simulink model "model_tmp_1p"  (R2015b)
settings: Solver=ode15s  StartTime=0.0  StopTime=T_sim  FixedStep=dt  RelTol=1e-3
PreLoadFcn:
  | setup_tmp_1p;
InitFcn:
  | setup_tmp_1p;
values from neighbouring files (symbols this model uses):
  A_act = [-100 0 0 0 0 -100 0 0 0 0 -100 0 ... (16 elements, 4x4)]    [CD_spline.mat]    (also in CL_spline.mat; setup.m = -100*eye(4); setup_tmp_1p.m = -100*eye(4); setup_tmp_4p.m = -100*eye(4))
  A_Kite = 7    [CD_spline.mat]    (also in CL_spline.mat; setup.m = 10.18; setup_tmp_1p.m = 10.18; setup_tmp_4p.m = 10.18)
  A_prd = [0 0 0 -640 0 0 0 0 0 0 -640 0 ... (36 elements, 6x6)]    [CD_spline.mat]    (also in CL_spline.mat; setup.m = 1000 * A_M_aug; setup_tmp_1p.m = 1000 * A_M_aug; setup_tmp_4p.m = 1000 * A_M_aug)
  A_ref = [0 0 0 -10000 0 0 0 0 0 0 -10000 0 ... (36 elements, 6x6)]    [CD_spline.mat]    (also in CL_spline.mat; setup.m = zeros(6); setup_tmp_1p.m = zeros(6); setup_tmp_4p.m = zeros(6))
  A_t_ref_cl = [0 0 0 -0.64 0 0 0 0 0 0 -0.64 0 ... (36 elements, 6x6)]    [CD_spline.mat]    (also in CL_spline.mat; setup.m = A_t_ref; setup_tmp_1p.m = A_t_ref; setup_tmp_4p.m = A_t_ref)
  ASideRel = 0    [CD_spline.mat]    (also in CL_spline.mat; setup.m; setup_tmp_1p.m; setup_tmp_4p.m)
  B_act = [100 0 0 0 0 100 0 0 0 0 100 0 ... (16 elements, 4x4)]    [CD_spline.mat]    (also in CL_spline.mat; setup.m = 100*eye(4); setup_tmp_1p.m = 100*eye(4); setup_tmp_4p.m = 100*eye(4))
  B_ref = [0 0 0 10000 0 0 0 0 0 0 10000 0 ... (18 elements, 6x3)]    [CD_spline.mat]    (also in CL_spline.mat; setup.m = zeros(6,3); setup_tmp_1p.m = zeros(6,3); setup_tmp_4p.m = zeros(6,3))
  B_t_ref_cl = [0 0 0 0.64 0 0 0 0 0 0 0.64 0 ... (18 elements, 6x3)]    [CD_spline.mat]    (also in CL_spline.mat)
  Bpbl = [0 0 0 1 0 0 0 0 0 0 1 0 ... (18 elements, 6x3)]    [CD_spline.mat]    (also in CL_spline.mat; setup.m = [zeros(3); eye(3)]; setup_tmp_1p.m = [zeros(3); eye(3)]; setup_tmp_4p.m = [zeros(3); eye(3)])
  c0 = 614000    [CD_spline.mat]    (also in CL_spline.mat; setup.m; setup_tmp_1p.m; setup_tmp_4p.m)
  C_A = [0 0.3 -1e-06 1 -0.3 0 1e-06 1 0 -0.3 -1e-06 1 ... (16 elements, 4x4)]    [CD_spline.mat]    (also in CL_spline.mat; setup.m = [0, -R, 0, R; setup_tmp_1p.m = [0, -R, 0, R; setup_tmp_4p.m = [0, -R, 0, R)
  C_A_inv = [0 -1.66666666667 -1.23358113847e-17 1.66666666667 1.66666666667 2.46716227694e-17 -1.66666666667 0 -250000 250000 -250000 250000 ... (16 elements, 4x4)]    [CD_spline.mat]    (also in CL_spline.mat; setup.m = C_A \eye(4); setup_tmp_1p.m = C_A \eye(4); setup_tmp_4p.m = C_A \eye(4))
  C_D_Kite = 0.05    [CD_spline.mat]    (also in CL_spline.mat; setup.m = 0.005; setup_tmp_1p.m = 0.005; setup_tmp_4p.m = 0.005)
  C_L_Kite = 0.1    [CD_spline.mat]    (also in CL_spline.mat; setup.m = 0.01; setup_tmp_1p.m = 0.01; setup_tmp_4p.m = 0.01)
  CD_tether = 0.96    [CD_spline.mat]    (also in CL_spline.mat; setup.m; setup_tmp_1p.m; setup_tmp_4p.m)
  d0 = 473    [CD_spline.mat]    (also in CL_spline.mat; setup.m; setup_tmp_1p.m; setup_tmp_4p.m)
  d_tether = 0.004    [CD_spline.mat]    (also in CL_spline.mat; setup.m; setup_tmp_1p.m; setup_tmp_4p.m)
  delta_dead = 0.5    [CD_spline.mat]    (also in CL_spline.mat; setup.m; setup_tmp_1p.m; setup_tmp_4p.m)
  e_0 = 0.01    [CD_spline.mat]    (also in CL_spline.mat; setup.m; setup_tmp_1p.m; setup_tmp_4p.m)
  epsilon = 0.6    [CD_spline.mat]    (also in CL_spline.mat; setup.m; setup_tmp_1p.m; setup_tmp_4p.m)
  eta_init = [0 0 0]    [CD_spline.mat]    (also in CL_spline.mat; setup.m = zeros(3,1); setup_tmp_1p.m = zeros(3,1); setup_tmp_4p.m = zeros(3,1))
  g = 9.81    [CD_spline.mat]    (also in CL_spline.mat; setup.m; setup_tmp_1p.m; setup_tmp_4p.m)
  g_vec = [0 0 9.81]    [CD_spline.mat]    (also in CL_spline.mat; setup.m = [0;0;9.81]; setup_tmp_1p.m = [0;0;9.81]; setup_tmp_4p.m = [0;0;9.81])
  Gamma_ad = 100    [CD_spline.mat]    (also in CL_spline.mat; setup.m = 100;100; setup_tmp_1p.m = 100;100; setup_tmp_4p.m = 100;100)
  Gamma_pred = 100    [CD_spline.mat]    (also in CL_spline.mat; setup.m; setup_tmp_1p.m; setup_tmp_4p.m)
  J = [0.018  0  0; 0  0.018  0; 0  0  0.009]    [CD_spline.mat]    (also in CL_spline.mat; setup.m = diag([Ixx, Iyy, Izz]); setup_tmp_1p.m = diag([Ixx, Iyy, Izz]); setup_tmp_4p.m = diag([Ixx, Iyy, Izz]))
  Jinv = [55.5555555556  0  0; 0  55.5555555556  0; 0  0  111.111111111]    [CD_spline.mat]    (also in CL_spline.mat; setup.m = J \ eye(3); setup_tmp_1p.m = J \ eye(3); setup_tmp_4p.m = J \ eye(3))
  k_e_eta = 10000    [CD_spline.mat]    (also in CL_spline.mat; setup.m; setup_tmp_1p.m; setup_tmp_4p.m)
  k_e_eta_dot = 400    [CD_spline.mat]    (also in CL_spline.mat; setup.m; setup_tmp_1p.m; setup_tmp_4p.m)
  k_e_eta_I = 1    [CD_spline.mat]    (also in CL_spline.mat; setup.m; setup_tmp_1p.m; setup_tmp_4p.m)
  K_i_t = [10  0  0; 0  10  0; 0  0  10]    [CD_spline.mat]    (also in CL_spline.mat; setup.m = 10*eye(3); setup_tmp_1p.m = 10*eye(3); setup_tmp_4p.m = 10*eye(3))
  K_v_t = [1.6  0  0; 0  1.6  0; 0  0  1.6]    [CD_spline.mat]    (also in CL_spline.mat; setup.m = 2*omega_0_trans*zeta_0_trans*eye(3); setup_tmp_1p.m = 2*omega_0_trans*zeta_0_trans*eye(3); setup_tmp_4p.m = 2*omega_0_trans*zeta_0_trans*eye(3))
  K_x_t = [0.64  0  0; 0  0.64  0; 0  0  0.64]    [CD_spline.mat]    (also in CL_spline.mat; setup.m = omega_0_trans^2*eye(3); setup_tmp_1p.m = omega_0_trans^2*eye(3); setup_tmp_4p.m = omega_0_trans^2*eye(3))
  l_s0 = 1    [CD_spline.mat]    (also in CL_spline.mat; setup.m = 1.42857142857; setup_tmp_1p.m = 1.42857142857; setup_tmp_4p.m = 2)
  m_kite = 7    [CD_spline.mat]    (also in CL_spline.mat; setup.m; setup_tmp_1p.m = 5;7; setup_tmp_4p.m = 6.21)
  m_p = 0.013    [CD_spline.mat]    (also in CL_spline.mat; setup.m = 0.0185714285714; setup_tmp_1p.m = 0.0185714285714; setup_tmp_4p.m = 0.026)
  m_uav = 3    [CD_spline.mat]    (also in CL_spline.mat; setup.m; setup_tmp_1p.m; setup_tmp_4p.m)
  n = 10    [CD_spline.mat]    (also in CL_spline.mat; setup.m; setup_tmp_1p.m; setup_tmp_4p.m)
  omega_init = [0 0 0]    [CD_spline.mat]    (also in CL_spline.mat; setup.m = zeros(3,1); setup_tmp_1p.m = zeros(3,1); setup_tmp_4p.m = zeros(3,1))
  p_init = [0 0 1 0 0 2 0 0 3 0 0 4 ... (30 elements, 30x1)]    [CD_spline.mat]    (also in CL_spline.mat; setup.m = zeros(3*n,1); setup_tmp_1p.m = zeros(3*n,1); setup_tmp_4p.m = zeros(3*n,1))
  P_prd = [712.5 0 0 156.25 0 0 0 712.5 0 0 156.25 0 ... (36 elements, 6x6)]    [CD_spline.mat]    (also in CL_spline.mat; setup.m = 1000 * P_tref; setup_tmp_1p.m = 1000 * P_tref; setup_tmp_4p.m = 1000 * P_tref)
  P_tref = [0.7125 0 0 0.15625 0 0 0 0.7125 0 0 0.15625 0 ... (36 elements, 6x6)]    [CD_spline.mat]    (also in CL_spline.mat; setup.m = lyap(A_M_aug', Q); setup_tmp_1p.m = lyap(A_M_aug', Q); setup_tmp_4p.m = lyap(A_M_aug', Q))
  rho_air = 1.225    [CD_spline.mat]    (also in CL_spline.mat; setup.m; setup_tmp_1p.m; setup_tmp_4p.m)
  rho_t = 0.013    [CD_spline.mat]    (also in CL_spline.mat; setup.m; setup_tmp_1p.m; setup_tmp_4p.m)
  sample_log = 0.01    [CD_spline.mat]    (also in CL_spline.mat; setup.m; setup_tmp_1p.m; setup_tmp_4p.m)
  t0 = 1    [CD_spline.mat]    (also in CL_spline.mat; setup.m; setup_tmp_1p.m; setup_tmp_4p.m)
  t1 = 3    [CD_spline.mat]    (also in CL_spline.mat; setup.m; setup_tmp_1p.m; setup_tmp_4p.m)
  T_launch = 40    [CD_spline.mat]    (also in CL_spline.mat; setup.m; setup_tmp_1p.m; setup_tmp_4p.m)
  Theta_max = 60    [CD_spline.mat]    (also in CL_spline.mat; setup.m; setup_tmp_1p.m; setup_tmp_4p.m)
  Thrust_Max = 80    [CD_spline.mat]    (also in CL_spline.mat; setup.m; setup_tmp_1p.m = 100; setup_tmp_4p.m = 1000000000)
  Tx = 10    [CD_spline.mat]    (also in CL_spline.mat; setup.m; setup_tmp_1p.m; setup_tmp_4p.m)
  Ty = 10    [CD_spline.mat]    (also in CL_spline.mat; setup.m; setup_tmp_1p.m; setup_tmp_4p.m)
  Tz = 10    [CD_spline.mat]    (also in CL_spline.mat; setup.m; setup_tmp_1p.m; setup_tmp_4p.m)
  v_w_vec = [1 1 1]    [CD_spline.mat]    (also in CL_spline.mat; setup.m = [1;0;0]; setup_tmp_1p.m = [1;0;0]; setup_tmp_4p.m = [1;0;0])
  x0num = 0    [CD_spline.mat]    (also in CL_spline.mat; polynomial_trajectory.m = double( solutions_x.x0 ))
  x1num = 0    [CD_spline.mat]    (also in CL_spline.mat; polynomial_trajectory.m = double( solutions_x.x1 ))
  x2num = 0    [CD_spline.mat]    (also in CL_spline.mat; polynomial_trajectory.m = double( solutions_x.x2 ))
  x3num = 0.05    [CD_spline.mat]    (also in CL_spline.mat; polynomial_trajectory.m = double( solutions_x.x3 ))
  x4num = -0.0075    [CD_spline.mat]    (also in CL_spline.mat; polynomial_trajectory.m = double( solutions_x.x4 ))
  x5num = 0.0003    [CD_spline.mat]    (also in CL_spline.mat; polynomial_trajectory.m = double( solutions_x.x5 ))
  x_drone_init = [0 0 10]    [CD_spline.mat]    (also in CL_spline.mat; setup.m = p_init(3*n-2:3*n); setup_KiteModel_4points.m = pos_UAV_init; setup_tmp_1p.m = p_init(3*n-2:3*n))
  xT = 5    [CD_spline.mat]    (also in CL_spline.mat; setup.m; setup_tmp_1p.m = 10; setup_tmp_4p.m = 10)
  y0num = 0    [CD_spline.mat]    (also in CL_spline.mat; polynomial_trajectory.m = double( solutions_y.y0 ))
  y1num = 0    [CD_spline.mat]    (also in CL_spline.mat; polynomial_trajectory.m = double( solutions_y.y1 ))
  y2num = 0    [CD_spline.mat]    (also in CL_spline.mat; polynomial_trajectory.m = double( solutions_y.y2 ))
  y3num = 0.1    [CD_spline.mat]    (also in CL_spline.mat; polynomial_trajectory.m = double( solutions_y.y3 ))
  y4num = -0.015    [CD_spline.mat]    (also in CL_spline.mat; polynomial_trajectory.m = double( solutions_y.y4 ))
  y5num = 0.0006    [CD_spline.mat]    (also in CL_spline.mat; polynomial_trajectory.m = double( solutions_y.y5 ))
  yT = 10    [CD_spline.mat]    (also in CL_spline.mat; setup.m; setup_tmp_1p.m = 0; setup_tmp_4p.m = 0)
  z0num = 10    [CD_spline.mat]    (also in CL_spline.mat; polynomial_trajectory.m = double( solutions_z.z0 ))
  z1num = 0    [CD_spline.mat]    (also in CL_spline.mat; polynomial_trajectory.m = double( solutions_z.z1 ))
  z2num = 0    [CD_spline.mat]    (also in CL_spline.mat; polynomial_trajectory.m = double( solutions_z.z2 ))
  z3num = 0.4    [CD_spline.mat]    (also in CL_spline.mat; polynomial_trajectory.m = double( solutions_z.z3 ))
  z4num = -0.06    [CD_spline.mat]    (also in CL_spline.mat; polynomial_trajectory.m = double( solutions_z.z4 ))
  z5num = 0.0024    [CD_spline.mat]    (also in CL_spline.mat; polynomial_trajectory.m = double( solutions_z.z5 ))
  zT = 50    [CD_spline.mat]    (also in CL_spline.mat; setup.m; setup_tmp_1p.m; setup_tmp_4p.m)
libraries: simulink x1
(part 1 of 2)
settings Model: Creator=Sebastian  LastModifiedBy=srapp
settings OptimizationCC: DefaultParameterBehavior=Inlined
settings DebuggingCC: MultiTaskRateTransMsg=warning
settings HardwareCC: ProdBitPerLong=64  ProdLargestAtomicFloat=None  ProdHWDeviceType=Intel->x86-64  TargetBitPerLong=64  TargetBitPerPointer=64  TargetIntDivRoundTo=Zero  TargetEndianess=LittleEndian  TargetWordSize=64  TargetHWDeviceType=Intel->x86-64
settings RTWCC: RTWCompilerOptimization=on
settings CodeAppCC: MaxIdLength=95

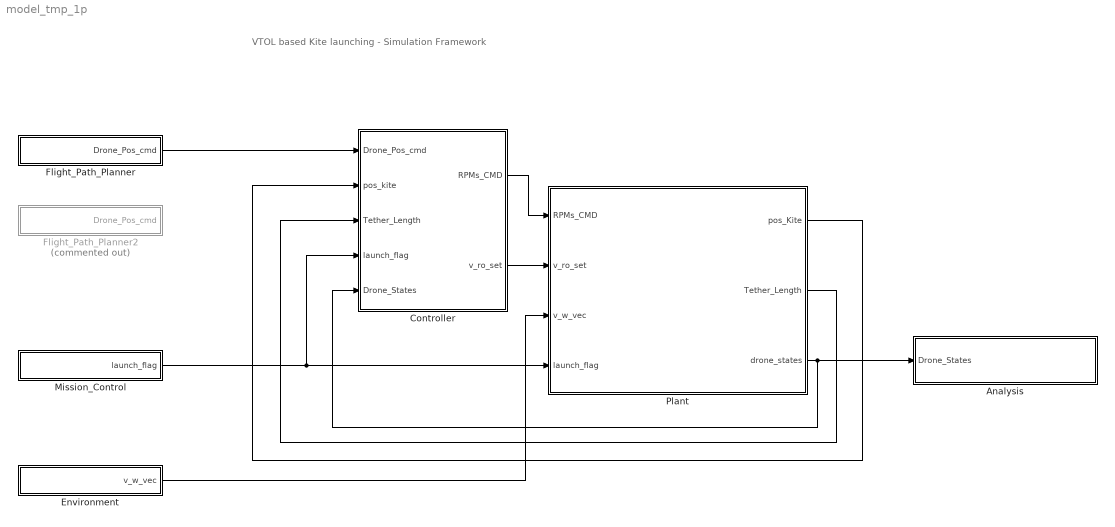
== system model_tmp_1p ==
  note: VTOL based Kite launching - Simulation Framework
  Analysis : Subsystem
  Controller : Subsystem
  Environment : Subsystem
  Flight_Path_Planner : Subsystem
  Flight_Path_Planner2 : Subsystem  Commented=on
  Mission_Control : Subsystem
  Plant : Subsystem
  wires:
  Flight_Path_Planner/1(Drone_Pos_cmd) -> Controller/1(Drone_Pos_cmd)
  Controller/1(RPMs_CMD) -> Plant/1(RPMs_CMD)
  Controller/2(v_ro_set) -> Plant/2(v_ro_set)
  Environment/1(v_w_vec) -> Plant/3(v_w_vec)
  Mission_Control/1(launch_flag) -> Plant/4(launch_flag), Controller/4(launch_flag)
  Plant/1(pos_Kite) -> Controller/2(pos_kite)
  Plant/2(Tether_Length) -> Controller/3(Tether_Length)
  Plant/3(drone_states) -> Controller/5(Drone_States), Analysis/1(Drone_States)

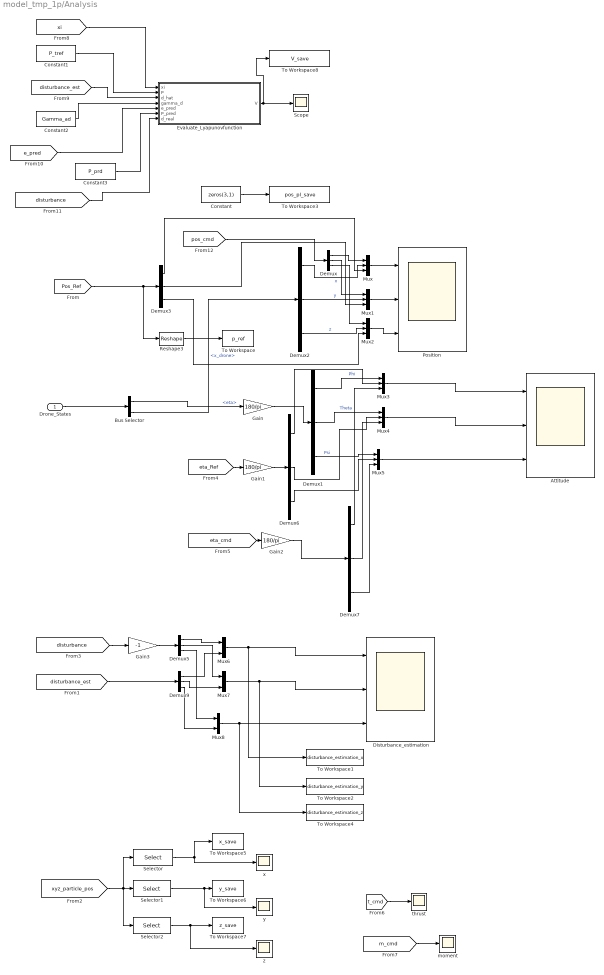
== system model_tmp_1p/Analysis ==
  Drone_States : Inport
  Attitude : Scope  NumInputPorts=3
  Bus Selector : BusSelector  OutputSignals=eta,x_drone
  Constant : Constant  Value=zeros(3,1)
  Constant1 : Constant  Value=P_tref
  Constant2 : Constant  Value=Gamma_ad
  Constant3 : Constant  Value=P_prd
  Demux{,1..3,5..7,9} (8 alike) : Demux  Outputs=3
  Disturbance_estimation : Scope  NumInputPorts=3
  Evaluate_Lyapunovfunction : MATLAB Function  TreatAsAtomicUnit=on
  Gain : Gain  Gain=180/pi
  Gain1 : Gain  Gain=180/pi
  Gain2 : Gain  Gain=180/pi
  Gain3 : Gain  Gain=-1
  Mux{,1..5} (6 alike) : Mux  Inputs=3
  Mux6 : Mux  Inputs=2
  Mux7 : Mux  Inputs=2
  Mux8 : Mux  Inputs=2
  Position : Scope  NumInputPorts=3
  Reshape3 : Reshape  OutputDimensionality=Column vector (2-D)
  Scope : Scope
  Selector : Selector  InputPortWidth=3*n  IndexOptions=Index vector (dialog)  Indices=[1 : 3 : 3*n-2]  OutputSizes=1
  Selector1 : Selector  InputPortWidth=3*n  IndexOptions=Index vector (dialog)  Indices=[2 : 3 : 3*n-1]  OutputSizes=1
  Selector2 : Selector  InputPortWidth=3*n  IndexOptions=Index vector (dialog)  Indices=[3 : 3 : 3*n]  OutputSizes=1
  To Workspace : ToWorkspace  VariableName=p_ref  SaveFormat=Timeseries  SampleTime=sample_log
  To Workspace1 : ToWorkspace  VariableName=disturbance_estimation_x  SaveFormat=Timeseries  SampleTime=sample_log
  To Workspace2 : ToWorkspace  VariableName=disturbance_estimation_y  SaveFormat=Timeseries  SampleTime=sample_log
  To Workspace3 : ToWorkspace  VariableName=pos_pl_save  SampleTime=sample_log
  To Workspace4 : ToWorkspace  VariableName=disturbance_estimation_z  SaveFormat=Timeseries  SampleTime=sample_log
  To Workspace5 : ToWorkspace  VariableName=x_save  SaveFormat=Timeseries  SampleTime=sample_log
  To Workspace6 : ToWorkspace  VariableName=y_save  SaveFormat=Timeseries  SampleTime=sample_log
  To Workspace7 : ToWorkspace  VariableName=z_save  SaveFormat=Timeseries  SampleTime=sample_log
  To Workspace8 : ToWorkspace  VariableName=V_save  SampleTime=sample_log
  moment : Scope
  thrust : Scope
  x : Scope
  y : Scope
  z : Scope
  wires:
  Bus Selector/1 -> Gain/1  "<eta>"
  Demux1/2 -> Mux4/1  "Theta"
  Demux1/3 -> Mux5/1  "Psi"
  Demux1/1 -> Mux3/1  "Phi"
  Demux2/2 -> Mux1/2  "y"
  Demux2/3 -> Mux2/2  "z"
  Demux2/1 -> Mux/2  "x"
  [pos_cmd] -> Demux/1
  Demux/1 -> Mux/1
  Mux/1 -> Position/1
  Demux/2 -> Mux1/1
  Mux1/1 -> Position/2
  Mux2/1 -> Position/3
  Demux/3 -> Mux2/1
  Bus Selector/2 -> Demux2/1  "<x_drone>"
  [Pos_Ref] -> Demux3/1, Reshape3/1
  Demux3/1 -> Mux/3
  Demux3/2 -> Mux1/3
  Demux3/3 -> Mux2/3
  Gain/1 -> Demux1/1
  [eta_Ref] -> Gain1/1
  Gain1/1 -> Demux6/1
  Mux3/1 -> Attitude/1
  Demux6/1 -> Mux3/2
  Demux6/2 -> Mux4/2
  Mux4/1 -> Attitude/2
  Demux6/3 -> Mux5/2
  Mux5/1 -> Attitude/3
  [eta_cmd] -> Gain2/1
  Demux7/1 -> Mux3/3
  Demux7/2 -> Mux4/3
  Demux7/3 -> Mux5/3
  Gain2/1 -> Demux7/1
  Constant/1 -> To Workspace3/1
  [disturbance] -> Gain3/1
  [disturbance_est] -> Demux9/1
  Mux6/1 -> To Workspace1/1, Disturbance_estimation/1
  Mux7/1 -> To Workspace2/1, Disturbance_estimation/2
  Mux8/1 -> To Workspace4/1, Disturbance_estimation/3
  Demux5/1 -> Mux6/1
  Demux5/2 -> Mux7/1
  Demux5/3 -> Mux8/1
  Demux9/1 -> Mux6/2
  Demux9/2 -> Mux7/2
  Demux9/3 -> Mux8/2
  Gain3/1 -> Demux5/1
  Selector/1 -> x/1, To Workspace5/1
  Selector1/1 -> y/1, To Workspace6/1
  Selector2/1 -> z/1, To Workspace7/1
  [xyz_particle_pos] -> Selector2/1, Selector/1, Selector1/1
  [t_cmd] -> thrust/1
  [m_cmd] -> moment/1
  Evaluate_Lyapunovfunction/1(V) -> To Workspace8/1, Scope/1
  [xi] -> Evaluate_Lyapunovfunction/1(xi)
  [disturbance_est] -> Evaluate_Lyapunovfunction/3(d_hat)
  Constant1/1 -> Evaluate_Lyapunovfunction/2(P)
  Constant2/1 -> Evaluate_Lyapunovfunction/4(gamma_d)
  [e_pred] -> Evaluate_Lyapunovfunction/5(e_pred)
  Constant3/1 -> Evaluate_Lyapunovfunction/6(P_pred)
  [disturbance] -> Evaluate_Lyapunovfunction/7(d_real)
  Reshape3/1 -> To Workspace/1
  Drone_States/1 -> Bus Selector/1

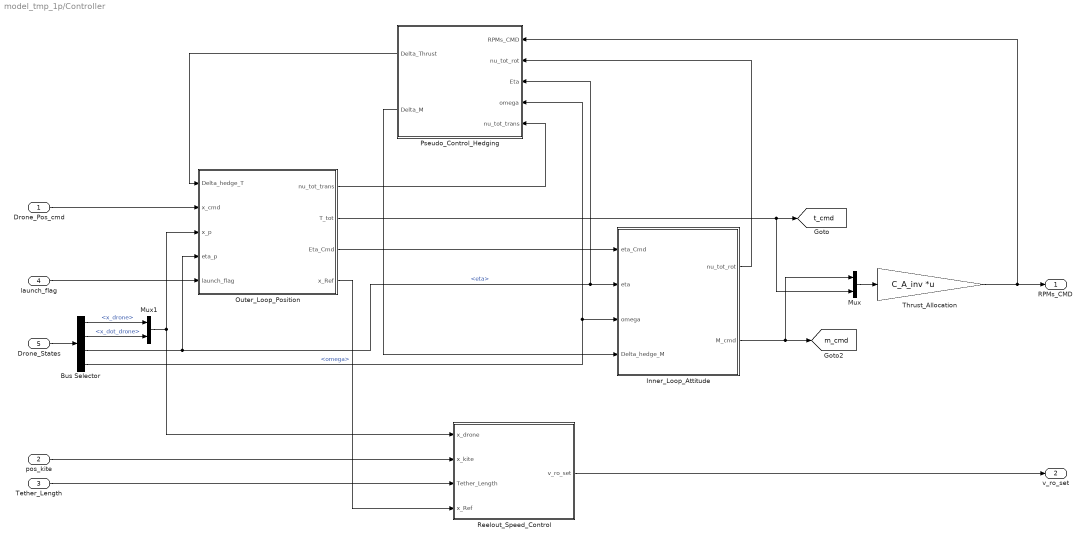
== system model_tmp_1p/Controller ==
  Drone_Pos_cmd : Inport
  pos_kite : Inport  Port=2
  Tether_Length : Inport  Port=3
  launch_flag : Inport  Port=4
  Drone_States : Inport  Port=5
  Bus Selector : BusSelector  OutputSignals=x_drone,x_dot_drone,eta,omega
  Inner_Loop_Attitude : Subsystem
  Mux : Mux  Inputs=2
  Mux1 : Mux  Inputs=2
  Outer_Loop_Position : Subsystem
  Pseudo_Control_Hedging : Subsystem
  Reelout_Speed_Control : Subsystem
  Thrust_Allocation : Gain  Gain=C_A_inv  Multiplication=Matrix(K*u)
  RPMs_CMD : Outport
  v_ro_set : Outport  Port=2
  tag scope: m_cmd=global, t_cmd=global
  wires:
  Drone_Pos_cmd/1 -> Outer_Loop_Position/2(x_cmd)
  Outer_Loop_Position/3(Eta_Cmd) -> Inner_Loop_Attitude/1(eta_Cmd)
  Reelout_Speed_Control/1(v_ro_set) -> v_ro_set/1
  pos_kite/1 -> Reelout_Speed_Control/2(x_kite)
  Tether_Length/1 -> Reelout_Speed_Control/3(Tether_Length)
  Outer_Loop_Position/4(x_Ref) -> Reelout_Speed_Control/4(x_Ref)
  launch_flag/1 -> Outer_Loop_Position/5(launch_flag)
  Mux/1 -> Thrust_Allocation/1
  Thrust_Allocation/1 -> Pseudo_Control_Hedging/1(RPMs_CMD), RPMs_CMD/1
  Outer_Loop_Position/2(T_tot) -> [t_cmd], Mux/2
  Inner_Loop_Attitude/2(M_cmd) -> [m_cmd], Mux/1
  Pseudo_Control_Hedging/1(Delta_Thrust) -> Outer_Loop_Position/1(Delta_hedge_T)
  Pseudo_Control_Hedging/2(Delta_M) -> Inner_Loop_Attitude/4(Delta_hedge_M)
  Outer_Loop_Position/1(nu_tot_trans) -> Pseudo_Control_Hedging/5(nu_tot_trans)
  Inner_Loop_Attitude/1(nu_tot_rot) -> Pseudo_Control_Hedging/2(nu_tot_rot)
  Drone_States/1 -> Bus Selector/1
  Bus Selector/3 -> Pseudo_Control_Hedging/3(Eta), Inner_Loop_Attitude/2(eta), Outer_Loop_Position/4(eta_p)  "<eta>"
  Bus Selector/4 -> Pseudo_Control_Hedging/4(omega), Inner_Loop_Attitude/3(omega)  "<omega>"
  Mux1/1 -> Reelout_Speed_Control/1(x_drone), Outer_Loop_Position/3(x_p)
  Bus Selector/1 -> Mux1/1  "<x_drone>"
  Bus Selector/2 -> Mux1/2  "<x_dot_drone>"

== system model_tmp_1p/Environment ==
  wind_vector : Constant  Value=v_w_vec
  v_w_vec : Outport
  wires:
  wind_vector/1 -> v_w_vec/1

== system model_tmp_1p/Flight_Path_Planner ==
  Clock : Clock
  Mux : Mux  Inputs=3
  Reference_Dynamic_x1 : MATLAB Function  TreatAsAtomicUnit=on
  Reference_Dynamic_x2 : MATLAB Function  TreatAsAtomicUnit=on
  Reference_Dynamic_x3 : MATLAB Function  TreatAsAtomicUnit=on
  Drone_Pos_cmd : Outport
  tag scope: pos_cmd=global
  wires:
  Mux/1 -> Drone_Pos_cmd/1, [pos_cmd]
  Reference_Dynamic_x2/1(z_ref) -> Mux/3
  Reference_Dynamic_x1/1(y_ref) -> Mux/2
  Clock/1 -> Reference_Dynamic_x1/1(t), Reference_Dynamic_x2/1(t), Reference_Dynamic_x3/1(t)
  Reference_Dynamic_x3/1(x_ref) -> Mux/1

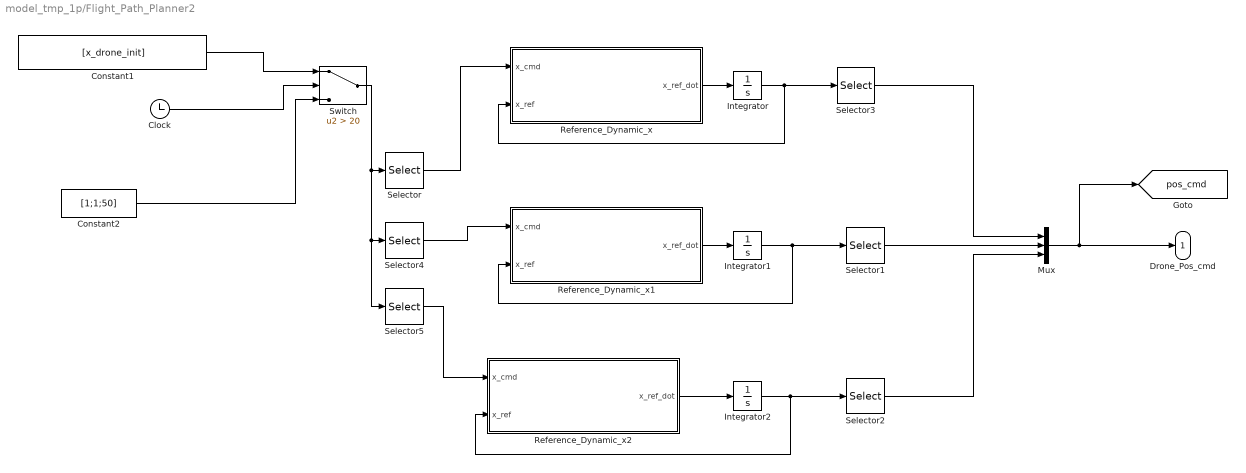
== system model_tmp_1p/Flight_Path_Planner2 ==
  Clock : Clock
  Constant1 : Constant  Value=[x_drone_init]
  Constant2 : Constant  Value=[1;1;50]
  Integrator : Integrator  InitialCondition=x_drone_init(1)
  Integrator1 : Integrator  InitialCondition=x_drone_init(2)
  Integrator2 : Integrator  InitialCondition=x_drone_init(3)
  Mux : Mux  Inputs=3
  Reference_Dynamic_x : MATLAB Function  TreatAsAtomicUnit=on
  Reference_Dynamic_x1 : MATLAB Function  TreatAsAtomicUnit=on
  Reference_Dynamic_x2 : MATLAB Function  TreatAsAtomicUnit=on
  Selector : Selector  InputPortWidth=3  IndexOptions=Index vector (dialog)  Indices=[1]  OutputSizes=1
  Selector1 : Selector  InputPortWidth=2  IndexOptions=Index vector (dialog)  Indices=[1]  OutputSizes=1
  Selector2 : Selector  InputPortWidth=2  IndexOptions=Index vector (dialog)  Indices=[1]  OutputSizes=1
  Selector3 : Selector  InputPortWidth=2  IndexOptions=Index vector (dialog)  Indices=[1]  OutputSizes=1
  Selector4 : Selector  InputPortWidth=3  IndexOptions=Index vector (dialog)  Indices=[2]  OutputSizes=1
  Selector5 : Selector  InputPortWidth=3  IndexOptions=Index vector (dialog)  Indices=[3]  OutputSizes=1
  Switch : Switch  Criteria=u2 > Threshold  Threshold=20
  Drone_Pos_cmd : Outport
  tag scope: pos_cmd=global
  wires:
  Switch/1 -> Selector/1, Selector4/1, Selector5/1
  Selector5/1 -> Reference_Dynamic_x2/1(x_cmd)
  Selector4/1 -> Reference_Dynamic_x1/1(x_cmd)
  Selector/1 -> Reference_Dynamic_x/1(x_cmd)
  Constant2/1 -> Switch/3
  Constant1/1 -> Switch/1
  Clock/1 -> Switch/2
  Integrator2/1 -> Selector2/1, Reference_Dynamic_x2/2(x_ref)
  Integrator1/1 -> Selector1/1, Reference_Dynamic_x1/2(x_ref)
  Selector2/1 -> Mux/3
  Selector1/1 -> Mux/2
  Selector3/1 -> Mux/1
  Integrator/1 -> Reference_Dynamic_x/2(x_ref), Selector3/1
  Reference_Dynamic_x/1(x_ref_dot) -> Integrator/1
  Reference_Dynamic_x2/1(x_ref_dot) -> Integrator2/1
  Reference_Dynamic_x1/1(x_ref_dot) -> Integrator1/1
  Mux/1 -> Drone_Pos_cmd/1, [pos_cmd]

== system model_tmp_1p/Mission_Control ==
  Clock : Clock
  Compare To Constant : simulink/Logic and Bit Operations/Compare To Constant  relop=>=  const=T_launch  OutDataTypeStr=boolean
  launch_flag : Outport
  wires:
  Clock/1 -> Compare To Constant/1
  Compare To Constant/1 -> launch_flag/1

== system model_tmp_1p/Plant ==
  RPMs_CMD : Inport
  v_ro_set : Inport  Port=2
  v_w_vec : Inport  Port=3
  launch_flag : Inport  Port=4
  Signal_Routing_1P1 : Subsystem
  Tether_Kite_Tether_UAV_Dynamics_1P : Subsystem
  pos_Kite : Outport
  Tether_Length : Outport  Port=2
  drone_states : Outport  Port=3  OutDataTypeStr=Bus: Drone_states
  wires:
  v_w_vec/1 -> Tether_Kite_Tether_UAV_Dynamics_1P/2(v_w_vec)
  v_ro_set/1 -> Tether_Kite_Tether_UAV_Dynamics_1P/3(v_ro_set)
  Tether_Kite_Tether_UAV_Dynamics_1P/3(l_tether) -> Tether_Length/1
  launch_flag/1 -> Tether_Kite_Tether_UAV_Dynamics_1P/4(launch_flag)
  RPMs_CMD/1 -> Tether_Kite_Tether_UAV_Dynamics_1P/1(RPMs)
  Tether_Kite_Tether_UAV_Dynamics_1P/1(x_dot) -> Signal_Routing_1P1/1(xdot_p)
  Tether_Kite_Tether_UAV_Dynamics_1P/2(x) -> Signal_Routing_1P1/2(x_p)
  Tether_Kite_Tether_UAV_Dynamics_1P/4(eta) -> Signal_Routing_1P1/3(eta)  "eta"
  Tether_Kite_Tether_UAV_Dynamics_1P/5(omega) -> Signal_Routing_1P1/4(omega)  "omega"
  Signal_Routing_1P1/1(pos_kite) -> pos_Kite/1
  Signal_Routing_1P1/2(Drone_States) -> drone_states/1

== system model_tmp_1p/Controller/Inner_Loop_Attitude ==
  eta_Cmd : Inport
  eta : Inport  Port=2
  omega : Inport  Port=3
  Delta_hedge_M : Inport  Port=4
  Add : Sum  Inputs=+-
  Add1 : Sum  Inputs=+-
  Add2 : Sum
  "P(I)D Error_Controller " : Subsystem
  Plant_Inversion_RD2 : Subsystem
  Reference_Model1 : Subsystem
  estimate_eta_dot : MATLAB Function  TreatAsAtomicUnit=on
  nu_tot_rot : Outport
  M_cmd : Outport  Port=2
  wires:
  eta/1 -> estimate_eta_dot/2(eta), Add/2, Plant_Inversion_RD2/3(Eta)
  Add/1 -> "P(I)D Error_Controller "/1(Eta_Error)  "e"
  Plant_Inversion_RD2/1(M_Cmd) -> M_cmd/1
  estimate_eta_dot/1(eta_dot) -> Add1/2, Plant_Inversion_RD2/2(Eta_Dot)
  Reference_Model1/2(Eta_Dot_R) -> Add1/1
  Reference_Model1/3(Nu_R) -> Add2/2
  Reference_Model1/1(Eta_R) -> Add/1
  Add1/1 -> "P(I)D Error_Controller "/2(Eta_Dot_Error)  "e_dot"
  "P(I)D Error_Controller "/1(u_error) -> Add2/1
  omega/1 -> estimate_eta_dot/1(omega), Plant_Inversion_RD2/1(omega)
  eta_Cmd/1 -> Reference_Model1/1(Eta_Cmd)
  Delta_hedge_M/1 -> Reference_Model1/2("Delta_hedge_M ")
  Add2/1 -> nu_tot_rot/1, Plant_Inversion_RD2/4(nu_tot)  "nu_tot"

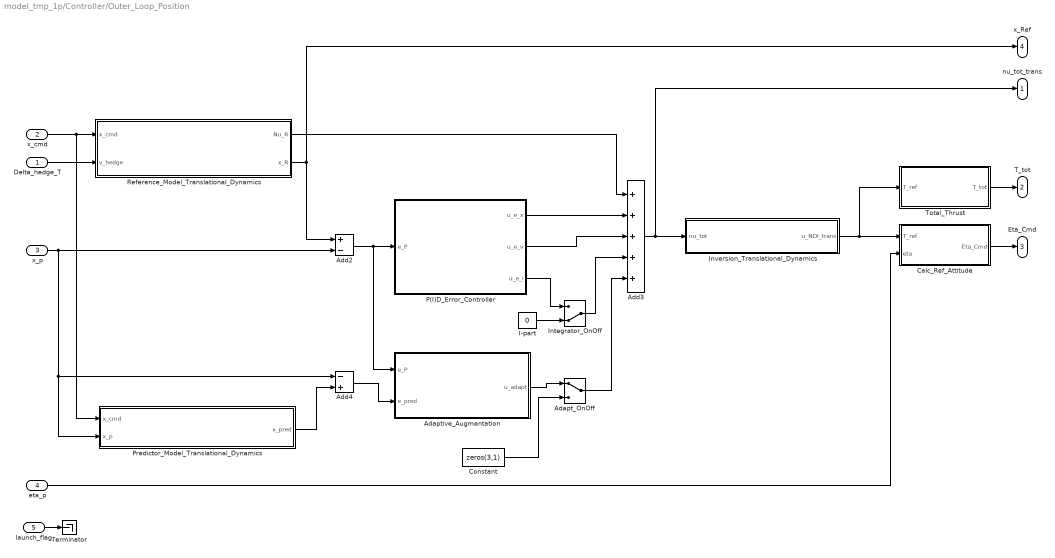
== system model_tmp_1p/Controller/Outer_Loop_Position ==
  Delta_hedge_T : Inport
  x_cmd : Inport  Port=2
  x_p : Inport  Port=3
  eta_p : Inport  Port=4
  launch_flag : Inport  Port=5
  Adapt_OnOff : ManualSwitch
  Adaptive_Augmentation : Subsystem
  Add2 : Sum  Inputs=+-
  Add3 : Sum  Inputs=+++++
  Add4 : Sum  Inputs=-+
  Calc_Ref_Attitude : MATLAB Function  TreatAsAtomicUnit=on
  Constant : Constant  Value=zeros(3,1)
  I-part : Constant  Value=0
  Integrator_OnOff : ManualSwitch  CurrentSetting=0
  Inversion_Translational_Dynamics : Subsystem
  P(I)D_Error_Controller : Subsystem
  Predictor_Model_Translational_Dynamics : Subsystem
  Reference_Model_Translational_Dynamics : Subsystem
  Terminator : Terminator
  Total_Thrust : MATLAB Function  TreatAsAtomicUnit=on
  nu_tot_trans : Outport
  T_tot : Outport  Port=2
  Eta_Cmd : Outport  Port=3  PortDimensions=[3,1]
  x_Ref : Outport  Port=4
  wires:
  eta_p/1 -> Calc_Ref_Attitude/2(eta)
  x_cmd/1 -> Predictor_Model_Translational_Dynamics/1(x_cmd), Reference_Model_Translational_Dynamics/1(x_cmd)
  Reference_Model_Translational_Dynamics/1(Nu_R) -> Add3/1
  x_p/1 -> Add2/2, Predictor_Model_Translational_Dynamics/2(x_p), Add4/1
  P(I)D_Error_Controller/1(u_e_x) -> Add3/2
  P(I)D_Error_Controller/2(u_e_v) -> Add3/3
  P(I)D_Error_Controller/3(u_e_i) -> Integrator_OnOff/1
  Adaptive_Augmentation/1(u_adapt) -> Adapt_OnOff/1
  Adapt_OnOff/1 -> Add3/5
  Constant/1 -> Adapt_OnOff/2
  Add4/1 -> Adaptive_Augmentation/2(e_pred)
  Predictor_Model_Translational_Dynamics/1(x_pred) -> Add4/2
  Calc_Ref_Attitude/1(Eta_Cmd) -> Eta_Cmd/1
  Integrator_OnOff/1 -> Add3/4
  I-part/1 -> Integrator_OnOff/2
  Reference_Model_Translational_Dynamics/2(x_R) -> Add2/1, x_Ref/1
  launch_flag/1 -> Terminator/1
  Add2/1 -> Adaptive_Augmentation/1(e_P), P(I)D_Error_Controller/1(e_P)
  Total_Thrust/1(T_tot) -> T_tot/1
  Delta_hedge_T/1 -> Reference_Model_Translational_Dynamics/2(v_hedge)
  Add3/1 -> nu_tot_trans/1, Inversion_Translational_Dynamics/1(nu_tot)
  Inversion_Translational_Dynamics/1(u_NDI_trans) -> Total_Thrust/1(T_ref), Calc_Ref_Attitude/1(T_ref)

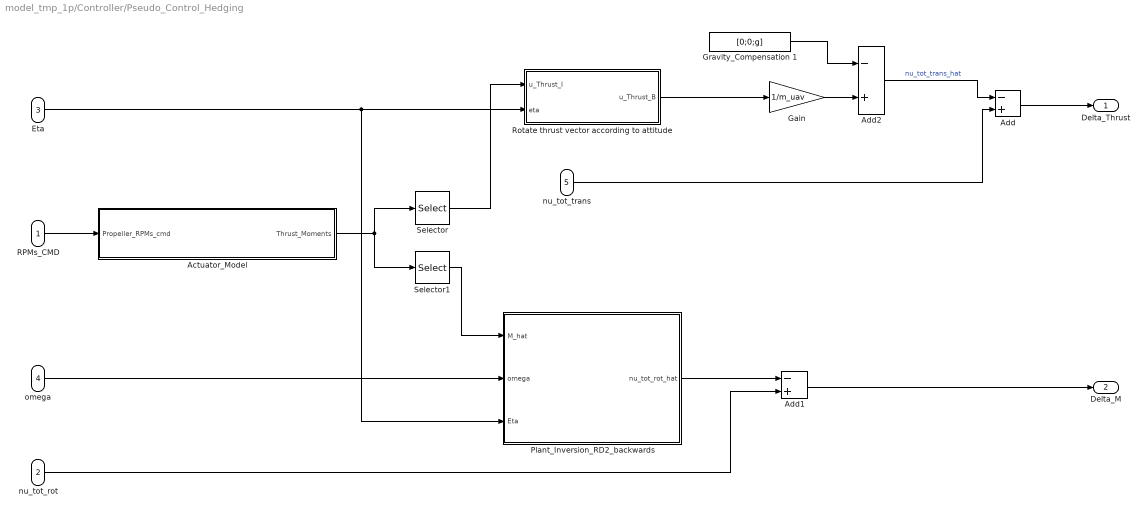
== system model_tmp_1p/Controller/Pseudo_Control_Hedging ==
  RPMs_CMD : Inport
  nu_tot_rot : Inport  Port=2
  Eta : Inport  Port=3
  omega : Inport  Port=4
  nu_tot_trans : Inport  Port=5
  Actuator_Model : Subsystem
  Add : Sum  Inputs=-+
  Add1 : Sum  Inputs=-+
  Add2 : Sum  Inputs=-+
  Gain : Gain  Gain=1/m_uav
  Gravity_Compensation 1 : Constant  Value=[0;0;g]
  Plant_Inversion_RD2_backwards : Subsystem
  Rotate thrust vector according to attitude : MATLAB Function  TreatAsAtomicUnit=on
  Selector : Selector  InputPortWidth=4  IndexOptions=Index vector (dialog)  Indices=[4]  OutputSizes=1
  Selector1 : Selector  InputPortWidth=4  IndexOptions=Index vector (dialog)  Indices=[1:3]  OutputSizes=1
  Delta_Thrust : Outport
  Delta_M : Outport  Port=2
  wires:
  Add/1 -> Delta_Thrust/1
  Selector/1 -> Rotate thrust vector according to attitude/1(u_Thrust_I)
  RPMs_CMD/1 -> Actuator_Model/1(Propeller_RPMs_cmd)
  nu_tot_trans/1 -> Add/2
  nu_tot_rot/1 -> Add1/2
  Selector1/1 -> Plant_Inversion_RD2_backwards/1(M_hat)
  Eta/1 -> Plant_Inversion_RD2_backwards/3(Eta), Rotate thrust vector according to attitude/2(eta)
  Add1/1 -> Delta_M/1
  Gravity_Compensation 1/1 -> Add2/1
  Rotate thrust vector according to attitude/1(u_Thrust_B) -> Gain/1
  Add2/1 -> Add/1  "nu_tot_trans_hat"
  Gain/1 -> Add2/2
  Actuator_Model/1(Thrust_Moments) -> Selector1/1, Selector/1
  omega/1 -> Plant_Inversion_RD2_backwards/2(omega)
  Plant_Inversion_RD2_backwards/1(nu_tot_rot_hat) -> Add1/1

== system model_tmp_1p/Controller/Reelout_Speed_Control ==
  note: UNDER CONSTRUCTION!
  x_drone : Inport
  x_kite : Inport  Port=2
  Tether_Length : Inport  Port=3
  x_Ref : Inport  Port=4
  Abs1 : Abs
  Activation_Function : MATLAB Function  TreatAsAtomicUnit=on
  Dot Product : DotProduct  InputSameDT=on  OutDataTypeStr=Inherit: Inherit via internal rule
  Gain1 : Gain  Gain=1000
  Product1 : Product
  Selector2 : Selector  InputPortWidth=6  IndexOptions=Index vector (dialog)  Indices=[1 2 3]  OutputSizes=1
  Sqrt : Sqrt  SaturateOnIntegerOverflow=on
  Subtract1 : Sum  Inputs=+-
  Terminator : Terminator
  Terminator2 : Terminator
  To Workspace5 : ToWorkspace  VariableName=safety_barrier  SaveFormat=Timeseries  SampleTime=sample_log
  v_ro_set : Outport
  wires:
  Dot Product/1 -> Sqrt/1
  Selector2/1 -> Dot Product/2, Dot Product/1
  x_Ref/1 -> Terminator2/1
  Tether_Length/1 -> Subtract1/2
  Subtract1/1 -> Activation_Function/1(d), Abs1/1, To Workspace5/1
  Gain1/1 -> v_ro_set/1
  x_kite/1 -> Terminator/1
  Activation_Function/1(safety_factor_vro) -> Product1/2
  Abs1/1 -> Product1/1
  Product1/1 -> Gain1/1
  Sqrt/1 -> Subtract1/1
  x_drone/1 -> Selector2/1

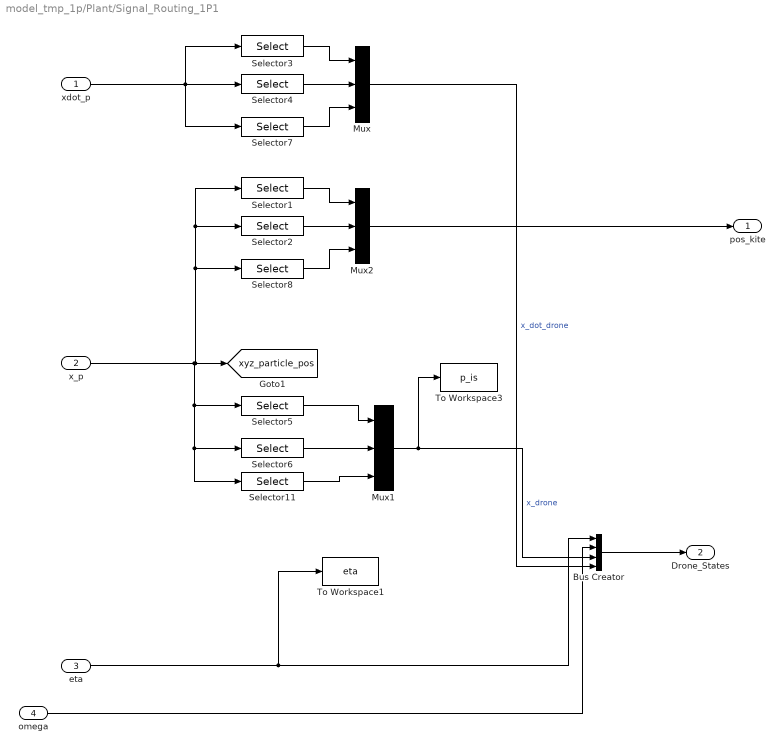
== system model_tmp_1p/Plant/Signal_Routing_1P1 ==
  xdot_p : Inport
  x_p : Inport  Port=2
  eta : Inport  Port=3
  omega : Inport  Port=4
  Bus Creator : BusCreator  Inputs=4  OutDataTypeStr=Bus: Drone_states
  Mux : Mux  Inputs=3
  Mux1 : Mux  Inputs=3
  Mux2 : Mux  Inputs=3
  Selector1 : Selector  InputPortWidth=3*n  IndexOptions=Index vector (dialog)  Indices=[3*(n-2)-2]  OutputSizes=1
  Selector11 : Selector  InputPortWidth=3*n  IndexOptions=Index vector (dialog)  Indices=[3*n]  OutputSizes=1
  Selector2 : Selector  InputPortWidth=3*n  IndexOptions=Index vector (dialog)  Indices=[3*(n-2)-1]  OutputSizes=1
  Selector3 : Selector  InputPortWidth=3*n  IndexOptions=Index vector (dialog)  Indices=[3*n-2]  OutputSizes=1
  Selector4 : Selector  InputPortWidth=3*n  IndexOptions=Index vector (dialog)  Indices=[3*n-1]  OutputSizes=1
  Selector5 : Selector  InputPortWidth=3*n  IndexOptions=Index vector (dialog)  Indices=[3*n-2]  OutputSizes=1
  Selector6 : Selector  InputPortWidth=3*n  IndexOptions=Index vector (dialog)  Indices=[3*n-1]  OutputSizes=1
  Selector7 : Selector  InputPortWidth=3*n  IndexOptions=Index vector (dialog)  Indices=[3*n]  OutputSizes=1
  Selector8 : Selector  InputPortWidth=3*n  IndexOptions=Index vector (dialog)  Indices=[3*(n-2)]  OutputSizes=1
  To Workspace1 : ToWorkspace  VariableName=eta  SaveFormat=Timeseries  SampleTime=sample_log
  To Workspace3 : ToWorkspace  VariableName=p_is  SaveFormat=Timeseries  SampleTime=sample_log
  pos_kite : Outport
  Drone_States : Outport  Port=2
  tag scope: xyz_particle_pos=global
  wires:
  Selector3/1 -> Mux/1
  Selector4/1 -> Mux/2
  Mux/1 -> Bus Creator/4  "x_dot_drone"
  Mux1/1 -> Bus Creator/3, To Workspace3/1  "x_drone"
  Selector5/1 -> Mux1/1
  Selector6/1 -> Mux1/2
  Selector7/1 -> Mux/3
  Selector11/1 -> Mux1/3
  x_p/1 -> Selector11/1, Selector6/1, Selector5/1, Selector1/1, Selector2/1, Selector8/1, [xyz_particle_pos]
  omega/1 -> Bus Creator/2
  eta/1 -> Bus Creator/1, To Workspace1/1
  Selector1/1 -> Mux2/1
  Selector2/1 -> Mux2/2
  Selector8/1 -> Mux2/3
  xdot_p/1 -> Selector7/1, Selector4/1, Selector3/1
  Mux2/1 -> pos_kite/1
  Bus Creator/1 -> Drone_States/1

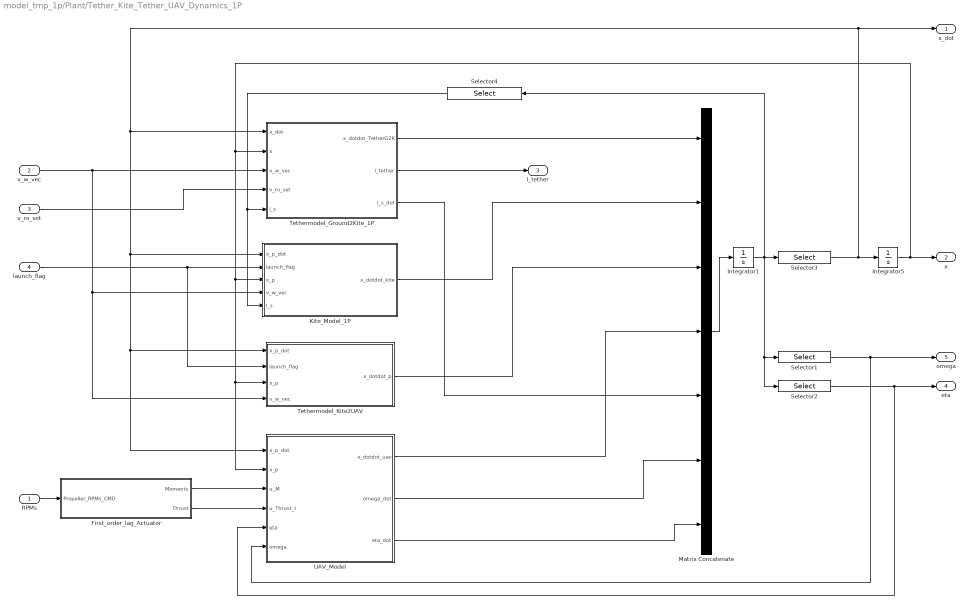
== system model_tmp_1p/Plant/Tether_Kite_Tether_UAV_Dynamics_1P ==
  RPMs : Inport
  v_w_vec : Inport  Port=2
  v_ro_set : Inport  Port=3
  launch_flag : Inport  Port=4
  First_order_lag_Actuator : Subsystem
  Integrator1 : Integrator  InitialCondition=[0*p_init;l_s0;omega_init;eta_init]
  Integrator5 : Integrator  InitialCondition=p_init
  Kite_Model_1P : Subsystem
  Matrix Concatenate : Concatenate  NumInputs=7  ConcatenateDimension=2
  Selector1 : Selector  InputPortWidth=3*n+1+6  IndexOptions=Index vector (dialog)  Indices=[3*n+2:3*n+4]  OutputSizes=1
  Selector2 : Selector  InputPortWidth=3*n+1+6  IndexOptions=Index vector (dialog)  Indices=[3*n+5:3*n+7]  OutputSizes=1
  Selector3 : Selector  InputPortWidth=3*n+1+6  IndexOptions=Index vector (dialog)  Indices=[1 : 3*n]  OutputSizes=1
  Selector4 : Selector  InputPortWidth=3*n+1+6  IndexOptions=Index vector (dialog)  Indices=[3*n+1:3*n+1]  OutputSizes=1
  Tethermodel_Ground2Kite_1P : Subsystem
  Tethermodel_Kite2UAV : Subsystem
  UAV_Model : Subsystem
  x_dot : Outport
  x : Outport  Port=2
  l_tether : Outport  Port=3
  eta : Outport  Port=4
  omega : Outport  Port=5
  wires:
  Matrix Concatenate/1 -> Integrator1/1
  Integrator1/1 -> Selector2/1, Selector1/1, Selector4/1, Selector3/1
  v_w_vec/1 -> Tethermodel_Ground2Kite_1P/3(v_w_vec), Tethermodel_Kite2UAV/4(v_w_vec), Kite_Model_1P/4(v_w_vec)
  launch_flag/1 -> Tethermodel_Kite2UAV/2(launch_flag), Kite_Model_1P/2(launch_flag)
  Kite_Model_1P/1(x_dotdot_kite) -> Matrix Concatenate/2
  Selector3/1 -> Integrator5/1, Tethermodel_Ground2Kite_1P/1(x_dot), UAV_Model/1(x_p_dot), Tethermodel_Kite2UAV/1(x_p_dot), Kite_Model_1P/1(x_p_dot), x_dot/1
  Integrator5/1 -> Tethermodel_Ground2Kite_1P/2(x), UAV_Model/2(x_p), Tethermodel_Kite2UAV/3(x_p), Kite_Model_1P/3(x_p), x/1
  v_ro_set/1 -> Tethermodel_Ground2Kite_1P/4(v_ro_set)
  Selector4/1 -> Tethermodel_Ground2Kite_1P/5(l_s), Kite_Model_1P/5(l_s)
  Tethermodel_Ground2Kite_1P/1(x_dotdot_TetherG2K) -> Matrix Concatenate/1
  Tethermodel_Ground2Kite_1P/2(l_tether) -> l_tether/1
  Tethermodel_Ground2Kite_1P/3(l_s_dot) -> Matrix Concatenate/5
  Tethermodel_Kite2UAV/1(x_dotdot_p) -> Matrix Concatenate/3
  UAV_Model/1(x_dotdot_uav) -> Matrix Concatenate/4
  UAV_Model/2(omega_dot) -> Matrix Concatenate/6
  UAV_Model/3(eta_dot) -> Matrix Concatenate/7
  Selector1/1 -> UAV_Model/6(omega), omega/1
  Selector2/1 -> UAV_Model/5(eta), eta/1
  RPMs/1 -> First_order_lag_Actuator/1(Propeller_RPMs_CMD)
  First_order_lag_Actuator/2(Thrust) -> UAV_Model/4(u_Thrust_I)
  First_order_lag_Actuator/1(Moments) -> UAV_Model/3(u_M)

== system model_tmp_1p/Controller/Inner_Loop_Attitude/P(I)D Error_Controller  ==
  Eta_Error : Inport
  Eta_Dot_Error : Inport  Port=2
  Add : Sum
  Gain : Gain  Gain=k_e_eta_dot
  Gain1 : Gain  Gain=k_e_eta
  Gain4 : Gain  Gain=k_e_eta_I
  Integrator2 : Integrator  InitialCondition=zeros(3,1)
  Terminator : Terminator
  u_error : Outport
  wires:
  Eta_Dot_Error/1 -> Gain/1
  Gain/1 -> Add/2
  Gain1/1 -> Add/1
  Add/1 -> u_error/1
  Eta_Error/1 -> Integrator2/1, Gain1/1  "e"
  Integrator2/1 -> Gain4/1
  Gain4/1 -> Terminator/1

== system model_tmp_1p/Controller/Inner_Loop_Attitude/Plant_Inversion_RD2 ==
  omega : Inport
  Eta_Dot : Inport  Port=2
  Eta : Inport  Port=3
  nu_tot : Inport  Port=4
  Constant1 : Constant  Value=J
  Plant_Inversion : MATLAB Function  TreatAsAtomicUnit=on
  M_Cmd : Outport
  wires:
  omega/1 -> Plant_Inversion/1(omega)
  Eta/1 -> Plant_Inversion/2(eta)
  Plant_Inversion/1(u_NDI) -> M_Cmd/1
  Constant1/1 -> Plant_Inversion/4(J)
  Eta_Dot/1 -> Plant_Inversion/3(eta_dot)
  nu_tot/1 -> Plant_Inversion/5(nu_tot)

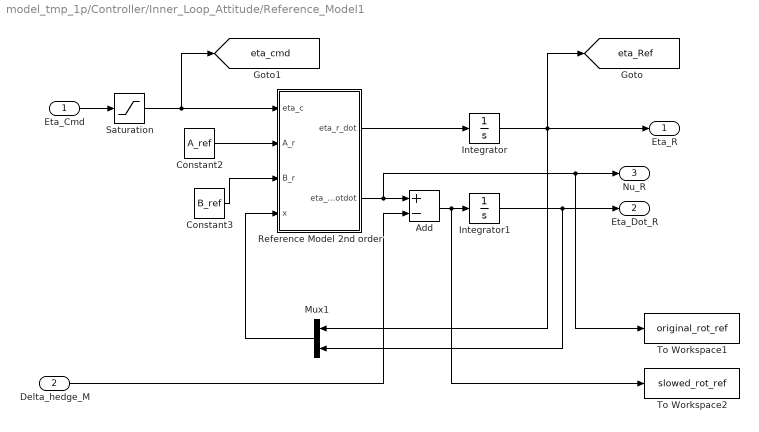
== system model_tmp_1p/Controller/Inner_Loop_Attitude/Reference_Model1 ==
  Eta_Cmd : Inport
  "Delta_hedge_M " : Inport  Port=2
  Add : Sum  Inputs=+-
  Constant2 : Constant  Value=A_ref
  Constant3 : Constant  Value=B_ref
  Integrator : Integrator  InitialCondition=zeros(3,1)
  Integrator1 : Integrator  InitialCondition=zeros(3,1)
  Mux1 : Mux  Inputs=2
  Reference Model 2nd order : MATLAB Function  TreatAsAtomicUnit=on
  Saturation : Saturate  UpperLimit=89*pi/180  LowerLimit=-89*pi/180
  To Workspace1 : ToWorkspace  VariableName=original_rot_ref  SaveFormat=Timeseries  SampleTime=sample_log
  To Workspace2 : ToWorkspace  VariableName=slowed_rot_ref  SaveFormat=Timeseries  SampleTime=sample_log
  Eta_R : Outport
  Eta_Dot_R : Outport  Port=2
  Nu_R : Outport  Port=3
  tag scope: eta_Ref=global, eta_cmd=global
  wires:
  Reference Model 2nd order/1(eta_r_dot) -> Integrator/1
  Reference Model 2nd order/2(eta_r_dotdot) -> To Workspace1/1, Nu_R/1, Add/1
  Integrator1/1 -> Eta_Dot_R/1, Mux1/2
  Mux1/1 -> Reference Model 2nd order/4(x)
  Constant2/1 -> Reference Model 2nd order/2(A_r)
  Constant3/1 -> Reference Model 2nd order/3(B_r)
  Integrator/1 -> Eta_R/1, [eta_Ref], Mux1/1
  Eta_Cmd/1 -> Saturation/1
  Saturation/1 -> [eta_cmd], Reference Model 2nd order/1(eta_c)
  "Delta_hedge_M "/1 -> Add/2
  Add/1 -> To Workspace2/1, Integrator1/1

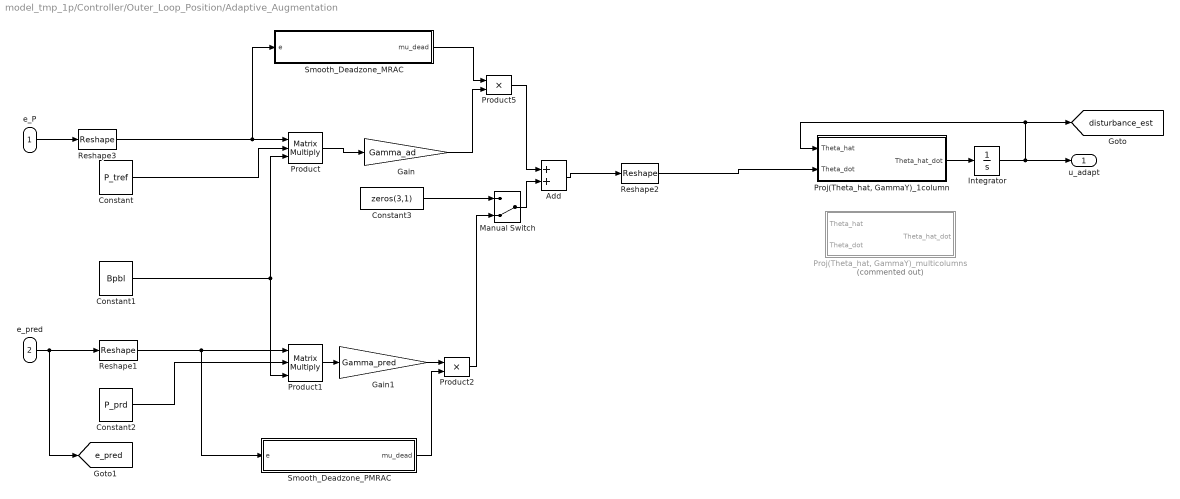
== system model_tmp_1p/Controller/Outer_Loop_Position/Adaptive_Augmentation ==
  e_P : Inport
  e_pred : Inport  Port=2
  Add : Sum
  Constant : Constant  Value=P_tref
  Constant1 : Constant  Value=Bpbl
  Constant2 : Constant  Value=P_prd
  Constant3 : Constant  Value=zeros(3,1)
  Gain : Gain  Gain=Gamma_ad
  Gain1 : Gain  Gain=Gamma_pred
  Integrator : Integrator  InitialCondition=zeros(3,1)
  Manual Switch : ManualSwitch  CurrentSetting=0
  Product : Product  Inputs=3  Multiplication=Matrix(*)
  Product1 : Product  Inputs=3  Multiplication=Matrix(*)
  Product2 : Product
  Product5 : Product
  "Proj(Theta_hat, GammaY)_1column" : Subsystem
  "Proj(Theta_hat, GammaY)_multicolumns" : Subsystem  Commented=on
  Reshape1 : Reshape  OutputDimensionality=Row vector (2-D)
  Reshape2 : Reshape  OutputDimensionality=Column vector (2-D)
  Reshape3 : Reshape  OutputDimensionality=Row vector (2-D)
  Smooth_Deadzone_MRAC : Subsystem
  Smooth_Deadzone_PMRAC : Subsystem
  u_adapt : Outport
  tag scope: disturbance_est=global, e_pred=global
  wires:
  e_P/1 -> Reshape3/1
  Constant1/1 -> Product/3, Product1/3
  Constant/1 -> Product/2
  Product/1 -> Gain/1
  e_pred/1 -> [e_pred], Reshape1/1
  Constant2/1 -> Product1/2
  Product1/1 -> Gain1/1
  Manual Switch/1 -> Add/2
  Constant3/1 -> Manual Switch/1
  Add/1 -> Reshape2/1
  Smooth_Deadzone_MRAC/1(mu_dead) -> Product5/1
  Gain/1 -> Product5/2
  Gain1/1 -> Product2/1
  Integrator/1 -> u_adapt/1, [disturbance_est], "Proj(Theta_hat, GammaY)_1column"/1(Theta_hat)
  "Proj(Theta_hat, GammaY)_1column"/1(Theta_hat_dot) -> Integrator/1
  Reshape2/1 -> "Proj(Theta_hat, GammaY)_1column"/2(Theta_dot)
  Product5/1 -> Add/1
  Product2/1 -> Manual Switch/2
  Reshape1/1 -> Product1/1, Smooth_Deadzone_PMRAC/1(e)
  Smooth_Deadzone_PMRAC/1(mu_dead) -> Product2/2
  Reshape3/1 -> Smooth_Deadzone_MRAC/1(e), Product/1

== system model_tmp_1p/Controller/Outer_Loop_Position/Inversion_Translational_Dynamics ==
  nu_tot : Inport
  Add1 : Sum
  Gain : Gain  Gain=m_uav
  Gravity_Compensation 1 : Constant  Value=[0;0;g]
  u_NDI_trans : Outport
  wires:
  Gain/1 -> u_NDI_trans/1
  Add1/1 -> Gain/1
  Gravity_Compensation 1/1 -> Add1/1
  nu_tot/1 -> Add1/2

== system model_tmp_1p/Controller/Outer_Loop_Position/P(I)D_Error_Controller ==
  e_P : Inport
  Integrator : Integrator
  K_e_v : Gain  Commented=on  Gain=K_v_t  Multiplication=Matrix(K*u)
  K_e_v1 : Gain  Commented=on  Gain=K_i_t  Multiplication=Matrix(K*u)
  K_e_v2 : Gain  Gain=5*K_v_t  Multiplication=Matrix(K*u)
  K_e_v3 : Gain  Gain=0.5*K_i_t  Multiplication=Matrix(K*u)
  K_e_x : Gain  Commented=on  Gain=K_x_t  Multiplication=Matrix(K*u)
  K_e_x1 : Gain  Gain=2*K_x_t  Multiplication=Matrix(K*u)
  Reshape : Reshape  OutputDimensionality=Column vector (2-D)
  Selector : Selector  InputPortWidth=6  IndexOptions=Index vector (dialog)  Indices=[1 2 3]  OutputSizes=1
  Selector1 : Selector  InputPortWidth=6  IndexOptions=Index vector (dialog)  Indices=[4 5 6]  OutputSizes=1
  u_e_x : Outport
  u_e_v : Outport  Port=2
  u_e_i : Outport  Port=3
  tag scope: xi=global
  wires:
  Selector/1 -> K_e_x1/1, K_e_v3/1
  K_e_v2/1 -> u_e_v/1
  K_e_x1/1 -> u_e_x/1
  K_e_v3/1 -> Integrator/1
  Integrator/1 -> u_e_i/1
  e_P/1 -> [xi], Reshape/1
  Selector1/1 -> K_e_v2/1
  Reshape/1 -> Selector1/1, Selector/1

== system model_tmp_1p/Controller/Outer_Loop_Position/Predictor_Model_Translational_Dynamics ==
  note: Wrong initialization?
  x_cmd : Inport
  x_p : Inport  Port=2
  Constant : Constant  Value=A_prd
  Constant1 : Constant  Value=B_t_ref_cl
  Constant3 : Constant  Value=A_t_ref_cl
  Integrator2 : Integrator  InitialCondition=zeros(6,1)
  Reference_Model_Position : MATLAB Function  TreatAsAtomicUnit=on
  Reshape1 : Reshape  OutputDimensionality=Row vector (2-D)
  x_pred : Outport
  wires:
  Reference_Model_Position/1(x_prd_dotdot) -> Integrator2/1
  Constant/1 -> Reference_Model_Position/1(A_prd)
  Constant1/1 -> Reference_Model_Position/3(B_ref)
  x_cmd/1 -> Reference_Model_Position/4(x_cmd)
  Integrator2/1 -> Reshape1/1, Reference_Model_Position/6(x_prd)
  Constant3/1 -> Reference_Model_Position/2(A_ref)
  x_p/1 -> Reference_Model_Position/5(x_p)
  Reshape1/1 -> x_pred/1

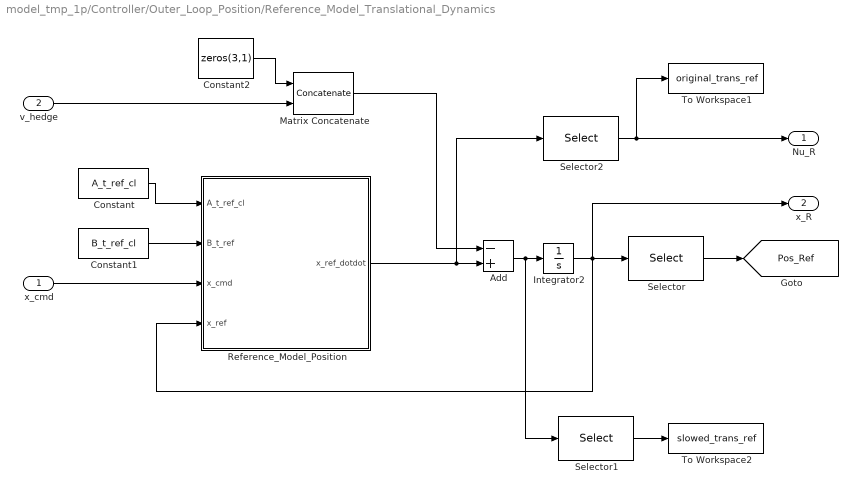
== system model_tmp_1p/Controller/Outer_Loop_Position/Reference_Model_Translational_Dynamics ==
  x_cmd : Inport
  v_hedge : Inport  Port=2
  Add : Sum  Inputs=-+
  Constant : Constant  Value=A_t_ref_cl
  Constant1 : Constant  Value=B_t_ref_cl
  Constant2 : Constant  Value=zeros(3,1)
  Integrator2 : Integrator  InitialCondition=[x_drone_init;zeros(3,1)]
  Matrix Concatenate : Concatenate  Mode=Multidimensional array
  Reference_Model_Position : MATLAB Function  TreatAsAtomicUnit=on
  Selector : Selector  InputPortWidth=6  IndexOptions=Index vector (dialog)  Indices=[1 2 3]  OutputSizes=1
  Selector1 : Selector  InputPortWidth=6  IndexOptions=Index vector (dialog)  Indices=[4 5 6]  OutputSizes=1
  Selector2 : Selector  InputPortWidth=6  IndexOptions=Index vector (dialog)  Indices=[4 5 6]  OutputSizes=1
  To Workspace1 : ToWorkspace  VariableName=original_trans_ref  SaveFormat=Timeseries  SampleTime=sample_log
  To Workspace2 : ToWorkspace  VariableName=slowed_trans_ref  SaveFormat=Timeseries  SampleTime=sample_log
  Nu_R : Outport
  x_R : Outport  Port=2
  tag scope: Pos_Ref=global
  wires:
  Reference_Model_Position/1(x_ref_dotdot) -> Selector2/1, Add/2
  Constant/1 -> Reference_Model_Position/1(A_t_ref_cl)
  Constant1/1 -> Reference_Model_Position/2(B_t_ref)
  x_cmd/1 -> Reference_Model_Position/3(x_cmd)
  Selector2/1 -> To Workspace1/1, Nu_R/1
  Selector/1 -> [Pos_Ref]
  Integrator2/1 -> Reference_Model_Position/4(x_ref), Selector/1, x_R/1
  v_hedge/1 -> Matrix Concatenate/2
  Matrix Concatenate/1 -> Add/1
  Add/1 -> Selector1/1, Integrator2/1
  Constant2/1 -> Matrix Concatenate/1
  Selector1/1 -> To Workspace2/1

== system model_tmp_1p/Controller/Pseudo_Control_Hedging/Actuator_Model ==
  Propeller_RPMs_cmd : Inport
  Gain : Gain  Gain=B_act  Multiplication=Matrix(K*u)
  Gain1 : Gain  Gain=A_act  Multiplication=Matrix(K*u)
  Integrator Limited1 : Integrator  InitialCondition=zeros(4,1)  LimitOutput=on  UpperSaturationLimit=Thrust_Max  LowerSaturationLimit=-Thrust_Max
  Output_Actuator : Gain  Gain=C_A  Multiplication=Matrix(K*u)
  Sum : Sum  Inputs=|++
  Thrust_Moments : Outport
  wires:
  Output_Actuator/1 -> Thrust_Moments/1
  Propeller_RPMs_cmd/1 -> Gain/1
  Gain/1 -> Sum/1
  Gain1/1 -> Sum/2
  Sum/1 -> Integrator Limited1/1
  Integrator Limited1/1 -> Output_Actuator/1, Gain1/1

== system model_tmp_1p/Controller/Pseudo_Control_Hedging/Plant_Inversion_RD2_backwards ==
  M_hat : Inport
  omega : Inport  Port=2
  Eta : Inport  Port=3
  Plant_Inversion : MATLAB Function  TreatAsAtomicUnit=on
  estimate_eta_dot : MATLAB Function  TreatAsAtomicUnit=on
  nu_tot_rot_hat : Outport
  wires:
  omega/1 -> estimate_eta_dot/1(omega), Plant_Inversion/1(omega)
  Eta/1 -> estimate_eta_dot/2(eta), Plant_Inversion/2(eta)
  Plant_Inversion/1(nu_tot_rot_hat) -> nu_tot_rot_hat/1
  M_hat/1 -> Plant_Inversion/4(M_hat)
  estimate_eta_dot/1(eta_dot) -> Plant_Inversion/3(eta_dot)

== system model_tmp_1p/Plant/Tether_Kite_Tether_UAV_Dynamics_1P/First_order_lag_Actuator ==
  Propeller_RPMs_CMD : Inport
  Actuator : Subsystem
  Selector : Selector  InputPortWidth=4  IndexOptions=Index vector (dialog)  Indices=[4]  OutputSizes=1
  Selector1 : Selector  InputPortWidth=4  IndexOptions=Index vector (dialog)  Indices=[1:3]  OutputSizes=1
  Moments : Outport
  Thrust : Outport  Port=2
  wires:
  Selector/1 -> Thrust/1
  Selector1/1 -> Moments/1
  Actuator/1(Thrust_Moments) -> Selector1/1, Selector/1
  Propeller_RPMs_CMD/1 -> Actuator/1(Propeller_RPMs_cmd)

== system model_tmp_1p/Plant/Tether_Kite_Tether_UAV_Dynamics_1P/Kite_Model_1P ==
  note: UNDER CONSTRUCTION!
  x_p_dot : Inport
  launch_flag : Inport  Port=2
  x_p : Inport  Port=3
  v_w_vec : Inport  Port=4
  l_s : Inport  Port=5
  Kite_Model : MATLAB Function  TreatAsAtomicUnit=on
  x_kite : Selector  InputPortWidth=3*n  IndexOptions=Index vector (dialog)  Indices=[3*(n-2)-2:3*(n-2)]  OutputSizes=1
  xdot_Kite : Selector  InputPortWidth=3*n  IndexOptions=Index vector (dialog)  Indices=[3*(n-2)-2:3*(n-2)]  OutputSizes=1
  xdot_aboveKite : Selector  InputPortWidth=3*n  IndexOptions=Index vector (dialog)  Indices=[3*(n-1)-2:3*(n-1)]  OutputSizes=1
  xdot_belowKite : Selector  InputPortWidth=3*n  IndexOptions=Index vector (dialog)  Indices=[3*(n-3)-2:3*(n-3)]  OutputSizes=1
  xp_aboveKite : Selector  InputPortWidth=3*n  IndexOptions=Index vector (dialog)  Indices=[3*(n-1)-2:3*(n-1)]  OutputSizes=1
  xp_belowKite : Selector  InputPortWidth=3*n  IndexOptions=Index vector (dialog)  Indices=[3*(n-3)-2:3*(n-3)]  OutputSizes=1
  x_dotdot_kite : Outport
  wires:
  xdot_aboveKite/1 -> Kite_Model/6(xdot_aboveKite)
  xdot_belowKite/1 -> Kite_Model/8(xdot_belowKite)
  x_kite/1 -> Kite_Model/4(x_kite)
  xp_belowKite/1 -> Kite_Model/5(xp_belowKite)
  xp_aboveKite/1 -> Kite_Model/3(xp_aboveKite)
  x_p_dot/1 -> xdot_aboveKite/1, xdot_Kite/1, xdot_belowKite/1
  xdot_Kite/1 -> Kite_Model/7(xdot_kite)
  launch_flag/1 -> Kite_Model/1(launch_flag)
  v_w_vec/1 -> Kite_Model/2(v_w_vec)
  x_p/1 -> xp_aboveKite/1, x_kite/1, xp_belowKite/1
  Kite_Model/1(x_dotdot_kite) -> x_dotdot_kite/1
  l_s/1 -> Kite_Model/9(l_s)

== system model_tmp_1p/Plant/Tether_Kite_Tether_UAV_Dynamics_1P/Tethermodel_Ground2Kite_1P ==
  x_dot : Inport
  x : Inport  Port=2
  v_w_vec : Inport  Port=3
  v_ro_set : Inport  Port=4
  l_s : Inport  Port=5
  Kite_p : Selector  InputPortWidth=3*n  IndexOptions=Index vector (dialog)  Indices=[3*(n-2)-2 : 3*(n-2)]  OutputSizes=1
  Kite_p1 : Selector  InputPortWidth=3*n  IndexOptions=Index vector (dialog)  Indices=[3*(n-2)-2 : 3*(n-2)]  OutputSizes=1
  Selector6 : Selector  InputPortWidth=3*n  IndexOptions=Index vector (dialog)  Indices=[1 : 3*(n-3)]  OutputSizes=1
  Tether_Ground2Kite : MATLAB Function  TreatAsAtomicUnit=on
  select_Tether_particles : Selector  InputPortWidth=3*n  IndexOptions=Index vector (dialog)  Indices=[1 : 3*(n-3)]  OutputSizes=1
  x_dotdot_TetherG2K : Outport
  l_tether : Outport  Port=2
  l_s_dot : Outport  Port=3
  wires:
  v_w_vec/1 -> Tether_Ground2Kite/3(v_w_vec)
  x_dot/1 -> Kite_p1/1, select_Tether_particles/1
  x/1 -> Kite_p/1, Selector6/1
  Tether_Ground2Kite/1(x_dotdot_TetherG2K) -> x_dotdot_TetherG2K/1
  Tether_Ground2Kite/2(l_tether) -> l_tether/1
  Tether_Ground2Kite/3(l_s_dot) -> l_s_dot/1
  l_s/1 -> Tether_Ground2Kite/5(l_s)
  v_ro_set/1 -> Tether_Ground2Kite/4(v_ro_set)
  select_Tether_particles/1 -> Tether_Ground2Kite/1(x_dot)
  Selector6/1 -> Tether_Ground2Kite/2(x)
  Kite_p1/1 -> Tether_Ground2Kite/7(xp_dot_kite)
  Kite_p/1 -> Tether_Ground2Kite/6(xp_kite)

== system model_tmp_1p/Plant/Tether_Kite_Tether_UAV_Dynamics_1P/Tethermodel_Kite2UAV ==
  x_p_dot : Inport
  launch_flag : Inport  Port=2
  x_p : Inport  Port=3
  v_w_vec : Inport  Port=4
  Tether_Kite2UAV : MATLAB Function  TreatAsAtomicUnit=on
  drone : Selector  InputPortWidth=3*n  IndexOptions=Index vector (dialog)  Indices=[3*n-2:3*n]  OutputSizes=1
  drone1 : Selector  InputPortWidth=3*n  IndexOptions=Index vector (dialog)  Indices=[3*n-2:3*n]  OutputSizes=1
  kite : Selector  InputPortWidth=3*n  IndexOptions=Index vector (dialog)  Indices=[3*(n-2)-2:3*(n-2)]  OutputSizes=1
  kite1 : Selector  InputPortWidth=3*n  IndexOptions=Index vector (dialog)  Indices=[3*(n-2)-2:3*(n-2)]  OutputSizes=1
  particle : Selector  InputPortWidth=3*n  IndexOptions=Index vector (dialog)  Indices=[3*(n-1)-2:3*(n-1)]  OutputSizes=1
  particle1 : Selector  InputPortWidth=3*n  IndexOptions=Index vector (dialog)  Indices=[3*(n-1)-2:3*(n-1)]  OutputSizes=1
  x_dotdot_p : Outport
  wires:
  Tether_Kite2UAV/1(x_dotdot_p) -> x_dotdot_p/1
  launch_flag/1 -> Tether_Kite2UAV/1(launch_flag)
  drone/1 -> Tether_Kite2UAV/2(xp_above)
  x_p_dot/1 -> drone1/1, kite1/1, particle1/1
  kite1/1 -> Tether_Kite2UAV/7(xp_dot_below)
  particle1/1 -> Tether_Kite2UAV/6(xp_dot)
  particle/1 -> Tether_Kite2UAV/3(xp)
  drone1/1 -> Tether_Kite2UAV/5(xp_dot_above)
  x_p/1 -> kite/1, particle/1, drone/1
  kite/1 -> Tether_Kite2UAV/4(xp_below)
  v_w_vec/1 -> Tether_Kite2UAV/8(v_w_vec)

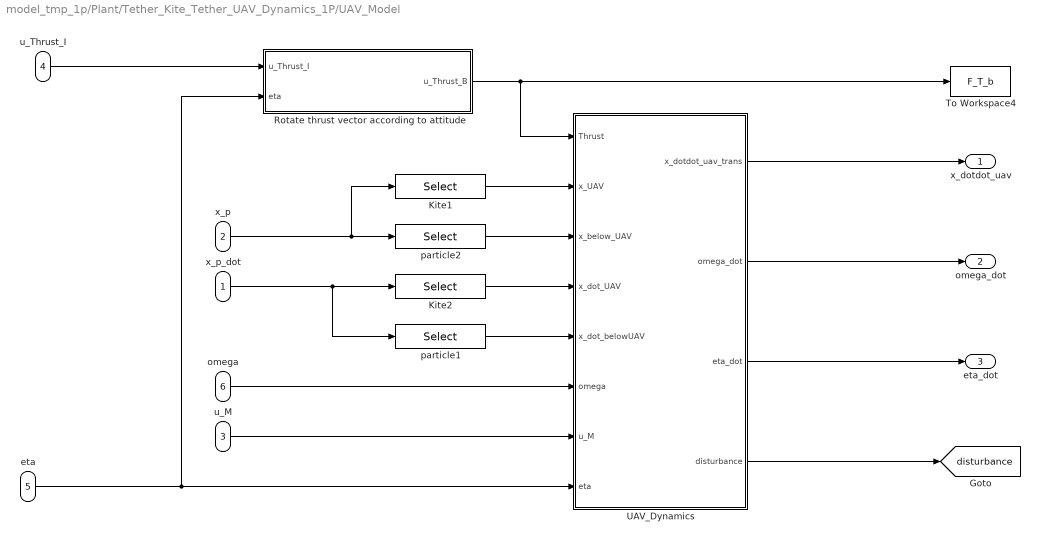
== system model_tmp_1p/Plant/Tether_Kite_Tether_UAV_Dynamics_1P/UAV_Model ==
  x_p_dot : Inport
  x_p : Inport  Port=2
  u_M : Inport  Port=3
  u_Thrust_I : Inport  Port=4
  eta : Inport  Port=5
  omega : Inport  Port=6
  Kite1 : Selector  InputPortWidth=3*n  IndexOptions=Index vector (dialog)  Indices=[3*n-2:3*n]  OutputSizes=1
  Kite2 : Selector  InputPortWidth=3*n  IndexOptions=Index vector (dialog)  Indices=[3*n-2:3*n]  OutputSizes=1
  Rotate thrust vector according to attitude : MATLAB Function  TreatAsAtomicUnit=on
  To Workspace4 : ToWorkspace  VariableName=F_T_b  SaveFormat=Timeseries  SampleTime=sample_log
  UAV_Dynamics : MATLAB Function  TreatAsAtomicUnit=on
  particle1 : Selector  InputPortWidth=3*n  IndexOptions=Index vector (dialog)  Indices=[3*(n-1)-2:3*(n-1)]  OutputSizes=1
  particle2 : Selector  InputPortWidth=3*n  IndexOptions=Index vector (dialog)  Indices=[3*(n-1)-2:3*(n-1)]  OutputSizes=1
  x_dotdot_uav : Outport
  omega_dot : Outport  Port=2
  eta_dot : Outport  Port=3
  tag scope: disturbance=global
  wires:
  Rotate thrust vector according to attitude/1(u_Thrust_B) -> To Workspace4/1, UAV_Dynamics/1(Thrust)
  UAV_Dynamics/1(x_dotdot_uav_trans) -> x_dotdot_uav/1
  Kite1/1 -> UAV_Dynamics/2(x_UAV)
  x_p/1 -> Kite1/1, particle2/1
  particle1/1 -> UAV_Dynamics/5(x_dot_belowUAV)
  Kite2/1 -> UAV_Dynamics/4(x_dot_UAV)
  x_p_dot/1 -> particle1/1, Kite2/1
  particle2/1 -> UAV_Dynamics/3(x_below_UAV)
  UAV_Dynamics/4(disturbance) -> [disturbance]
  UAV_Dynamics/2(omega_dot) -> omega_dot/1
  UAV_Dynamics/3(eta_dot) -> eta_dot/1
  u_M/1 -> UAV_Dynamics/7(u_M)
  eta/1 -> Rotate thrust vector according to attitude/2(eta), UAV_Dynamics/8(eta)
  omega/1 -> UAV_Dynamics/6(omega)
  u_Thrust_I/1 -> Rotate thrust vector according to attitude/1(u_Thrust_I)
